simulink model "EAF_single_phase"  (R2025b)
settings: Solver=FixedStepAuto  StartTime=0.0  StopTime=1  RelTol=1e-3
model workspace (MAT data in the model file):
  GateChoice = "linear"
values from neighbouring files (symbols this model uses):
  Ts_meas = 0.005    [ctrlSys.sldd]
libraries: fl_lib x1, eeRmsMeasurement x1, nesl_utility x1, ee_lib x1
settings Model: DataDictionary=ctrlSys.sldd  Creator=LYG  LastModifiedBy=A

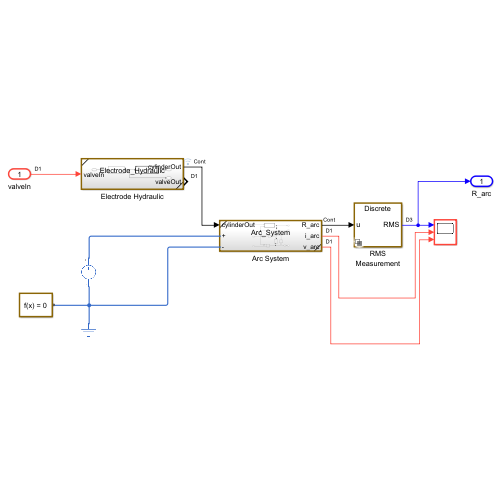
[thumbnail: Simulink's stored preview of the top-level diagram]
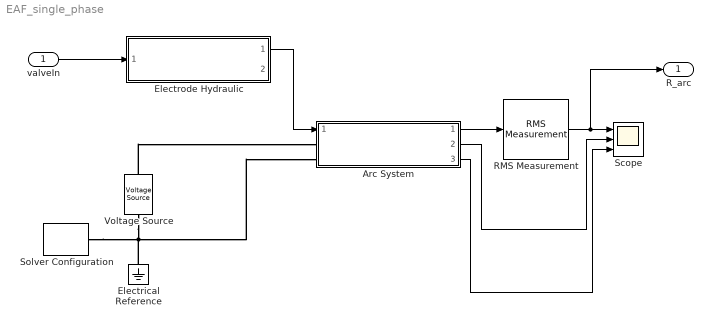
== system EAF_single_phase ==
  valveIn : Inport
  Arc System : Subsystem  ReferencedSubsystem=Arc_System
  Electrical Reference : fl_lib/Electrical/Electrical Elements/Electrical Reference
  Electrode Hydraulic : Subsystem  ReferencedSubsystem=Electrode_Hydraulic
  RMS Measurement : eeRmsMeasurement/RMS Measurement  LabelModeActiveChoice=Total  F=f  SpecifyHarmonics=off  K=[0 1 2]  Ts=Ts_meas
      settings: LibrarySourceBlock=|
      | ee_sl_lib/Measurements/RMS
      | Measurement
  Scope : Scope  NumInputPorts=3
      settings: ActiveDisplayYMinimum=-0.0050446440276730124  ActiveDisplayYMaximum=0.045401796249057116
  Solver Configuration : nesl_utility/Solver Configuration  PhysicalDomain=network_engine_domain  SubClassName=solver  LeftPortType=input  RightPortType=generic  Tones=[]  Harmonics=[]  SimulateNoise=off  Profile=off  UseLocalSampling=off  EnableSwitchedLinearOptims=on  FrequencyDomain=off  UseCCode=off  RelTol=0.001  AbsTol=0.001  MinStep=1e-09  ToWorkspace=off  RevertToSquareIcSolve=off  NumHomotopyIterations=100  PhasorMode=off  PhasorModeNumHarmonics=1  ConsistencySolver=NEWTON_XTOL_AFTER_FTOL  IndexReductionMethod=DerivativeReplacement  DoDC=off  ResidualTolerance=1e-09  ConsistencyTolSource=GLOBAL  ConsistencyAbsTol=0.001  ConsistencyRelTol=0.001  ConsistencyTolFactor=0.001  UseLocalSolver=on  LocalSolverChoice=NE_BACKWARD_EULER_ADVANCER  ResolveIndetEquations=on  FunctionEvalNumThread=1  LocalSolverSampleTime=Ts_local  DoFixedCost=off  MaxNonlinIter=3  MaxModeIter=2  ComputeImpulses=off  ImpulseIterations=2  LinearAlgebra=auto  LinearAlgebraNumThread=0  EquationFormulation=NE_TIME_EF  DelaysMemoryBudget=1024  AutomaticFiltering=on  FilteringTimeConstant=0.001  PartitionStorageMethod=AS_NEEDED  PartitionMemoryBudget=1024  PartitionMethod=ROBUST  MultibodyUseLocalSolver=off  MultibodyLocalSolverChoice=ODE1  MultibodyLocalSolverSampleTime=0.001
  Voltage Source : ee_lib/Sources/Voltage Source  dc_voltage=0 V  ac_voltage=sqrt(2) * 580 V  ac_shift=0 rad  ac_frequency=f Hz  noise_mode=ee.enum.sources.noise.Disabled  PSD=0 V^2/Hz  sample_time=1e-3 s  repeatability=ee.enum.sources.repeatability.NotRepeatable  user_seed=0  auto_seed=4111000739  i_specify=off  i_priority=None  i=0 A  i_nominal_specify=off  i_nominal_value=1  i_nominal_unit=A  v_specify=off  v_priority=None  v=0 V  v_nominal_specify=off  v_nominal_value=1  v_nominal_unit=V
  R_arc : Outport
  wires:
  Arc System/1 -> RMS Measurement/1
  RMS Measurement/1 -> R_arc/1, Scope/1
  Arc System/2 -> Scope/2
  Arc System/3 -> Scope/3
  Electrode Hydraulic/1 -> Arc System/1
  valveIn/1 -> Electrode Hydraulic/1
  connections:
  Voltage Source/LConn1 -- Arc System/LConn1
  Voltage Source/RConn1 -- Electrical Reference/LConn1 -- Solver Configuration/RConn1 -- Arc System/LConn2
